simulink model "controller_comb_sim"  (R2020a)
settings: Solver=FixedStepAuto  StartTime=0.0  StopTime=options.T_train  FixedStep=0.005  RelTol=1e-3
values from neighbouring files (symbols this model uses):
  ss1 = ss(K1)    [lpv_config.m]
  ss2 = ss(K2)    [lpv_config.m]
  sysP = ss(P)    [lpv_config.m]
undefined symbols (not defined in the file or in its folder): options
libraries: simulink x3
settings Model: Creator=kekatos  LastModifiedBy=kekatos
settings DataIOCC: SignalLogging=off  DSMLogging=off  ReturnWorkspaceOutputs=off

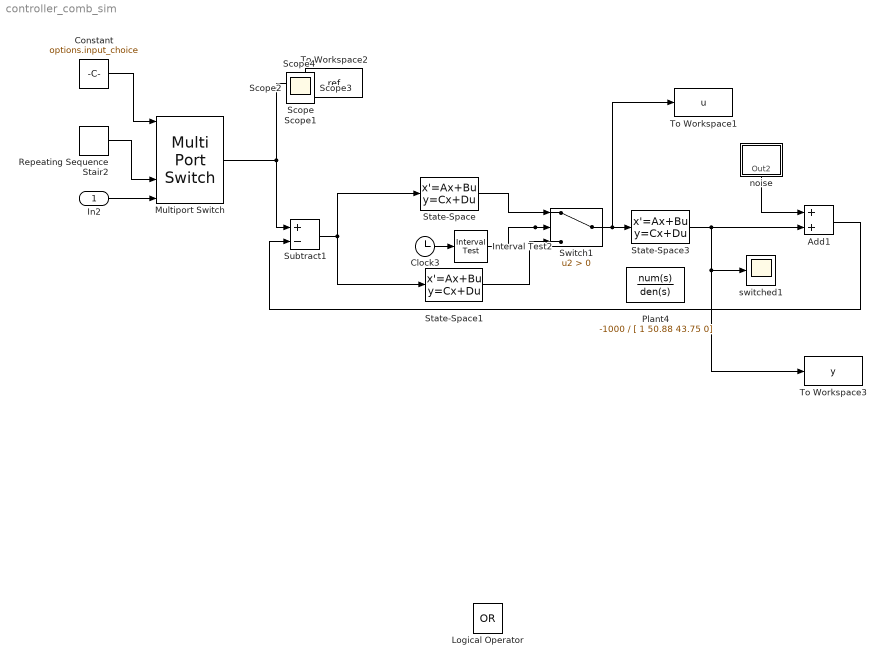
== system controller_comb_sim ==
  In2 : Inport
  Add1 : Sum
  Clock3 : Clock
  Constant : Constant  Value=options.input_choice
  Interval Test2 : simulink/Logic and Bit Operations/Interval Test  IntervalClosedRight=on  uplimit=options.T_train  IntervalClosedLeft=on  lowlimit=options.T_train/2  OutDataTypeStr=boolean
  Logical Operator : Logic  Operator=OR  AllPortsSameDT=off  OutDataTypeStr=boolean
  Multiport Switch : MultiPortSwitch  Inputs=4
  Plant4 : TransferFcn  Numerator=-1000  Denominator=[ 1 50.88 43.75 0]
  Repeating Sequence Stair2 : simulink/Sources/Repeating Sequence Stair  OutValues=options.sim_cov  tsamp=options.ref_Ts  OutMin=[]  OutMax=[]  OutDataTypeStr=double  OutputDataTypeScalingMode=double  OutDataType=fixdt(0,8)  ConRadixGroup=Best Precision: Vector-wise  OutScaling=2^-12
  State-Space : StateSpace  A=ss1.A  B=ss1.B  C=ss1.C  D=ss1.D  InitialCondition=0
  State-Space1 : StateSpace  A=ss2.A  B=ss2.B  C=ss2.C  D=ss2.D  InitialCondition=0
  State-Space3 : StateSpace  A=sysP.A  B=sysP.B  C=sysP.C  D=sysP.D  InitialCondition=0
  Subtract1 : Sum  Inputs=+-
  Switch1 : Switch  Criteria=u2 > Threshold
  To Workspace1 : ToWorkspace  VariableName=u  SaveFormat=Structure With Time  SampleTime=options.dt
  To Workspace2 : ToWorkspace  VariableName=ref  SaveFormat=Structure With Time  SampleTime=options.dt
  To Workspace3 : ToWorkspace  VariableName=y  SaveFormat=Structure With Time  SampleTime=options.dt
  noise : Subsystem
  switched1 : Scope
  Scope{,1..4} (5 alike) : Scope
  wires:
  Switch1/1 -> State-Space3/1, To Workspace1/1
  Interval Test2/1 -> Switch1/2
  Multiport Switch/1 -> Subtract1/1, To Workspace2/1
  Add1/1 -> Subtract1/2
  State-Space3/1 -> switched1/1, To Workspace3/1, Add1/2
  State-Space1/1 -> Switch1/3
  State-Space/1 -> Switch1/1
  Subtract1/1 -> State-Space1/1, State-Space/1
  ? -> ?
  Clock3/1 -> Interval Test2/1
  noise/1(Out2) -> Add1/1
  Constant/1 -> Multiport Switch/1
  Repeating Sequence Stair2/1 -> Multiport Switch/4
  In2/1 -> Multiport Switch/5

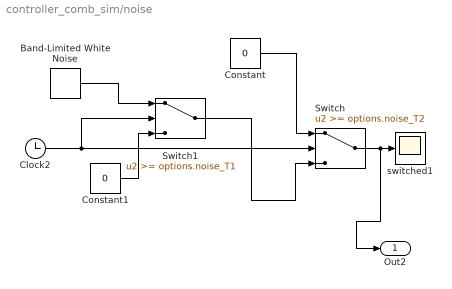
== system controller_comb_sim/noise ==
  Band-Limited White Noise : simulink/Sources/Band-Limited White Noise  Cov=1e-8  Ts=options.dt  seed=randi(1000)
  Clock2 : Clock
  Constant : Constant  Value=0
  Constant1 : Constant  Value=0
  Switch : Switch  Threshold=options.noise_T2
  Switch1 : Switch  Threshold=options.noise_T1
  switched1 : Scope
  Out2 : Outport
  wires:
  Clock2/1 -> Switch1/2, Switch/2
  Constant/1 -> Switch/1
  Constant1/1 -> Switch1/3
  Band-Limited White Noise/1 -> Switch1/1
  Switch/1 -> Out2/1, switched1/1
  Switch1/1 -> Switch/3
